simulink model "SimCodeGen_mfun_model"  (R2023b)
settings: Solver=VariableStepAuto  StartTime=0.0  StopTime=10.0  RelTol=1e-3
values from neighbouring files (symbols this model uses):
  params = [ig c s ms CA CM]    [init_DSMS.m]    (also in init_DSMS_vorlage.m = [m c d g]; init_elast_Getriebe.m = [ig c s ms C_A_S C_M_S d]; init_inv.m = [m1 m2 l1 l2 s1 s2 C_1_S g d1 d2 m A_P B_P ig C_M]; init_inverse_pendel.m = [m1 m2 l1 l2 s1 s2 C_1_S g ig C_M_S])
  x1_ic = zeros(4,1)    [init_DSMS.m]    (also in init_DSMS_vorlage.m = zeros(2,1); init_elast_Getriebe.m; init_inv.m; init_inverse_pendel.m)
settings Model: Creator=Flo  LastModifiedBy=Flo

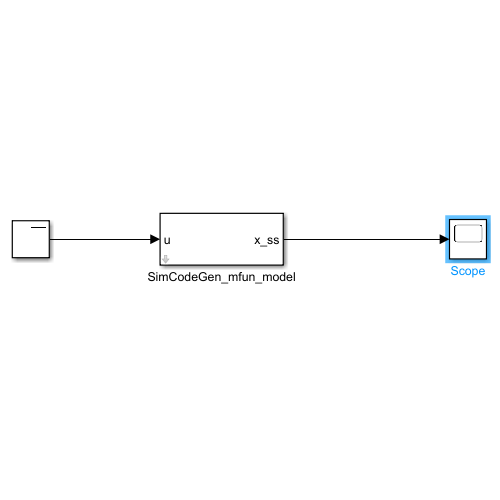
[thumbnail: Simulink's stored preview of the top-level diagram]
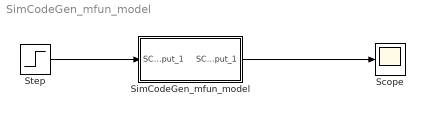
== system SimCodeGen_mfun_model ==
  Scope : Scope
  SimCodeGen_mfun_model : Subsystem  mask{SC_param_0=params, SC_x1_ic=x1_ic}
      mask prompts: SC_param_0 "params"
      mask Display:
      | port_label('input', 1, 'u');
      | port_label('output', 1, 'x_ss');
  Step : Step  After=5  SampleTime=0
  wires:
  Step/1 -> SimCodeGen_mfun_model/1(SC_input_1)
  SimCodeGen_mfun_model/1(SC_output_1) -> Scope/1

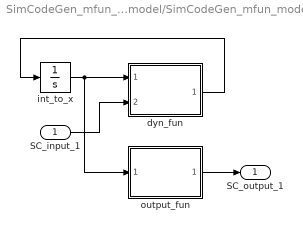
== system SimCodeGen_mfun_model/SimCodeGen_mfun_model ==
  SC_input_1 : Inport
  dyn_fun : MATLAB Function  TreatAsAtomicUnit=on
  int_to_x : Integrator  InitialCondition=[SC_x1_ic]
  output_fun : MATLAB Function  TreatAsAtomicUnit=on
  SC_output_1 : Outport
  wires:
  output_fun/1(SC_output_0) -> SC_output_1/1
  int_to_x/1 -> dyn_fun/1(SC_state), output_fun/1(SC_state)
  SC_input_1/1 -> dyn_fun/2(SC_input_0)
  dyn_fun/1(SC_state_dot) -> int_to_x/1

== matlab function SimCodeGen_mfun_model/dyn_fun ==
  data: SC_state input size=[4]; SC_state_dot output size=[4]; SC_input_0 input size=[1]; SC_param_0 parameter
function SC_state_dot  = dyn_fun(SC_state, SC_input_0, SC_param_0)
    SC_state_dot = zeros(4, 1);
    SC_state_x_0 = SC_state(1:4);
    SC_eval = zeros(4,1);
    SC_eval(1) = SC_state_x_0(3);
    SC_eval(2) = SC_state_x_0(4);
    t1 = 0.1e1 / CM;
    t2 = SC_param_0(1);
    t6 = SC_input_0(1) / t2 * t1;
    t7 = t2 ^ 2;
    t9 = SC_state_x_0(2) * SC_param_0(2);
    t12 = t1 / t7;
    SC_eval(3) = t12 * t9 + t6;
    t16 = SC_param_0(3) ^ 2;
    t17 = t16 * ms;
    SC_eval(4) = -t6 - (CM * t7 + CA + t17) * t12 / (t17 + CA) * t9;
    SC_state_dot(1:4) = SC_eval(1:4);
end

== matlab function SimCodeGen_mfun_model/output_fun ==
  data: SC_state input size=[4]; SC_output_0 output size=[4]; SC_param_0 parameter size=[6]
function SC_output_0  = y_fun(SC_state, SC_param_0)
    SC_output_0 = zeros(4,1);
    SC_state_x_0 = SC_state(1:4);
    SC_output_0(1) = SC_state_x_0(1);
    SC_output_0(2) = SC_state_x_0(2);
    SC_output_0(3) = SC_state_x_0(3);
    SC_output_0(4) = SC_state_x_0(4);
end
